simulink model "recordMotion"  (R2019b)
settings: Solver=FixedStepDiscrete  StartTime=0.0  StopTime=inf  FixedStep=1/100  RelTol=1e-3
libraries: simulink x1, simulink_extras x1, xpcrtudplib x1, xpcutilitieslib x1
settings Model: EnablePacing=on  Creator=Aljaz  LastModifiedBy=Aljaz
settings DataIOCC: SaveOutput=off  SaveTime=off  ReturnWorkspaceOutputs=off

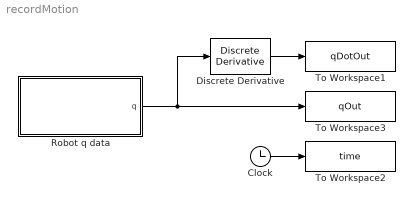
== system recordMotion ==
  Clock : Clock
  Discrete Derivative : simulink/Discrete/Discrete Derivative  gainval=1.0  ICPrevScaledInput=0.0  OutMin=[]  OutMax=[]  OutDataType=fixdt(1, 16)  OutScaling=2^-10  DoSatur=off
  Robot q data : Subsystem
  To Workspace1 : ToWorkspace  VariableName=qDotOut  SampleTime=-1
  To Workspace2 : ToWorkspace  VariableName=time  SampleTime=-1
  To Workspace3 : ToWorkspace  VariableName=qOut  SampleTime=-1
  wires:
  Robot q data/1(q) -> To Workspace3/1, Discrete Derivative/1
  Clock/1 -> To Workspace2/1
  Discrete Derivative/1 -> To Workspace1/1

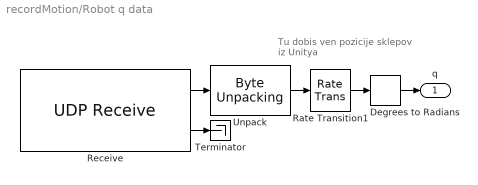
== system recordMotion/Robot q data ==
  note: Tu dobis ven pozicije sklepov iz Unitya
  Degrees to Radians : simulink_extras/Transformations/Degrees to Radians
  Rate Transition1 : RateTransition
  Receive : xpcrtudplib/UDP Receive  ipAddressVal=Use host-target connection  localPort=25106  rcvWidth=7*4  rcvFmAny=off  fmAddress=127.0.0.1  rcvMulticast=off  multicastAddress={}  maxUDPQueue=8  sampleTime=0.01
      settings: SourceProductName=Simulink Real-Time
  Terminator : Terminator
  Unpack : xpcutilitieslib/Byte Unpacking   MaskUnpackedDataTypes={'single'}  MaskUnpackedDataSizes={[7]}  MaskAlignment=1
      settings: SourceProductName=Simulink Real-Time  SourceProductBaseCode=XP
  q : Outport
  wires:
  Unpack/1 -> Rate Transition1/1
  Receive/1 -> Unpack/1
  Receive/2 -> Terminator/1
  Rate Transition1/1 -> Degrees to Radians/1
  Degrees to Radians/1 -> q/1
